simulink model "A_ASK"  (Simulink 10.1)
settings: Solver=VariableStepDiscrete  StartTime=0.0  StopTime=sim_t  RelTol=1e-3  EnableMultiTasking=on
values from neighbouring files (symbols this model uses):
  A1a = 0.5    [TP1.m]
  A2a = 2    [TP1.m]
undefined symbols (not defined in the file or in its folder): A3a, BSTa, PZa, STa
libraries: commrandsrc2 x1, dsparch4 x1
settings Model: Creator=usuario  LastModifiedBy=Fer
settings DataIOCC: LimitDataPoints=on  SignalLoggingSaveFormat=ModelDataLogs
settings OptimizationCC: ExpressionDepthLimit=2147483647  InitFltsAndDblsToZero=on
settings DebuggingCC: SaveWithParameterizedLinksMsg=none  SignalResolutionControl=TryResolveAllWithWarning  SolverPrmCheckMsg=warning  MultiTaskDSMMsg=warning  MultiTaskCondExecSysMsg=none  FcnCallInpInsideContextMsg=warning  StateNameClashWarn=warning
settings SFSimCC: SimParseCustomCode=off
settings GRTTargetCC: TargetFcnLib=ansi_tfl_tmw.mat

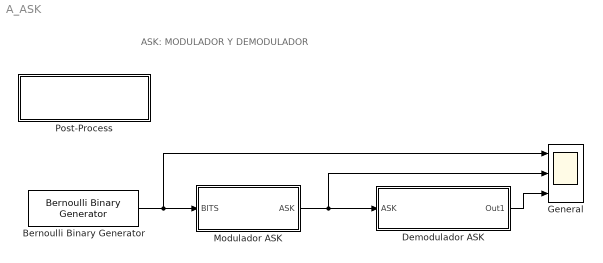
== system A_ASK ==
  note: ASK: MODULADOR Y DEMODULADOR
  Bernoulli Binary Generator : commrandsrc2/Bernoulli Binary Generator  P=PZa  seed=81  Ts=BSTa  frameBased=off  sampPerFrame=1  orient=off  outDataType=double
      settings: SourceProductBaseCode=CM
  Demodulador ASK : Subsystem
  General : Scope  NumInputPorts=3
  Modulador ASK : Subsystem
  Post-Process : Subsystem  mask{sim_t=100, BSTa=5, FFa=5, A1a=.5, A2a=2}
      mask prompts: sim_t "Sim Time [100]"; BSTa "Source Sample Time"; FFa "Freq. factor [1]"; A1a "Mod - Amp Sine 1 [2]"; A2a "Mod - Amp Sine 2 [.5]"
      mask init:
      | %sim_t = 100; %simulation time
      | %BST = 5; % source sample time
      | PZa = .4; % probability of zero
      | %ST = 1/20; % sample time
      | %SxP = 50; % samples per period
      | %A1 = 2; % amplitude sine 1 - mod.
      | %A2 = .5; % amplitude sine 2 - mod.
      | A3a = 1; % amplitude sine 3 - demod.
      | 
      | switch sim_t
      |     case 1
      |         sim_t = 50;
      |     case 2
      |         sim_t = 100;
      |     case 3
      |         sim_t = 250;
      |     case 4
      |         sim_t = 500;
      |     case 5
      |         sim_t = 1000;        
      | end
      | 
      | % Sample Time Source Configure
      | switch BSTa
      |     case 1
      |         BSTa = 5;
      |     case 2
      |         BSTa = 8;
      |     case 3
      |         BSTa = 10;
      |     case 4
      |         BSTa = 12;        
      | end
      | 
      | STa=(1/BSTa*1/4)*1/FFa;
      | %SxP=50*1/FF;
      | SxPa=(BSTa*10);
      | 
      | assignin('base','sim_t', sim_t );
      | assignin('base','FFa', FFa );
      | assignin('base','BSTa', BSTa );
      | assignin('base','PZa', PZa );
      | assignin('base','STa', STa );
      | assignin('base','SxPa', SxPa );
      | assignin('base','A1a', A1a );
      | assignin('base','A2a', A2a );
      | assignin('base','A3a', A3a );
      mask TypeOptions sim_t: 50 | 100 | 250 | 500 | 1000
      mask TypeOptions BSTa: 5 | 8 | 10 | 12
      mask Display: disp('Sim Parameters')
  wires:
  Bernoulli Binary Generator/1 -> Modulador ASK/1(BITS), General/1
  Modulador ASK/1(ASK) -> Demodulador ASK/1(ASK), General/2
  Demodulador ASK/1(Out1) -> General/3

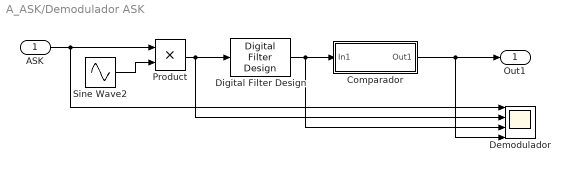
== system A_ASK/Demodulador ASK ==
  ASK : Inport
  Comparador : Subsystem
  Demodulador : Scope  NumInputPorts=4
  Digital Filter Design : dsparch4/Digital Filter Design  mwdsp_browser_bugfix_var=off
  Product : Product  RndMeth=Zero
  Sine Wave2 : Sin  SineType=Sample based  Amplitude=A3a  Frequency=2*10*pi  Samples=SxPa  SampleTime=STa
  Out1 : Outport
  wires:
  ASK/1 -> Demodulador/1, Product/1
  Sine Wave2/1 -> Product/2
  Product/1 -> Digital Filter Design/1, Demodulador/2
  Digital Filter Design/1 -> Demodulador/3, Comparador/1(In1)
  Comparador/1(Out1) -> Demodulador/4, Out1/1

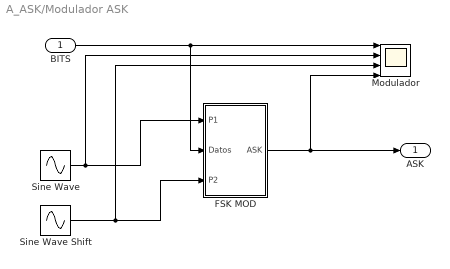
== system A_ASK/Modulador ASK ==
  BITS : Inport
  FSK MOD : Subsystem
  Modulador : Scope  NumInputPorts=4
  Sine Wave : Sin  SineType=Sample based  Amplitude=A1a  Frequency=2*10*pi  Samples=SxPa  SampleTime=STa
  Sine Wave Shift : Sin  SineType=Sample based  Amplitude=A2a  Frequency=2*10*pi  Phase=-pi  Samples=SxPa  SampleTime=STa
  ASK : Outport
  wires:
  BITS/1 -> Modulador/1, FSK MOD/2(Datos)
  Sine Wave/1 -> Modulador/2, FSK MOD/1(P1)
  Sine Wave Shift/1 -> Modulador/3, FSK MOD/3(P2)
  FSK MOD/1(ASK) -> Modulador/4, ASK/1

== system A_ASK/Post-Process ==

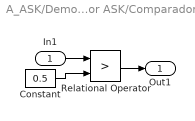
== system A_ASK/Demodulador ASK/Comparador ==
  In1 : Inport
  Constant : Constant  Value=0.5
  Relational Operator : RelationalOperator  Operator=>  OutDataTypeStr=boolean  RndMeth=Nearest
  Out1 : Outport
  wires:
  Constant/1 -> Relational Operator/2
  In1/1 -> Relational Operator/1
  Relational Operator/1 -> Out1/1

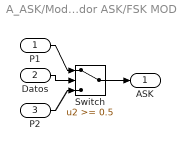
== system A_ASK/Modulador ASK/FSK MOD ==
  P1 : Inport
  Datos : Inport  Port=2
  P2 : Inport  Port=3
  Switch : Switch  Threshold=0.5
  ASK : Outport
  wires:
  P1/1 -> Switch/1
  Datos/1 -> Switch/2
  Switch/1 -> ASK/1
  P2/1 -> Switch/3
